simulink model "pmsm_summer_last"  (R2014a)
settings: Solver=ode23t  StartTime=0.0  StopTime=3  RelTol=1e-3
undefined symbols (not defined in the file or in its folder): sigbuilder_block
libraries: powerlib x6, powerlib_extras x3, simulink x1
settings Model: Creator=Andrew  LastModifiedBy=Administrator
settings DataIOCC: SignalLoggingSaveFormat=ModelDataLogs
settings OptimizationCC: ExpressionDepthLimit=2147483647
settings DebuggingCC: UnderspecifiedInitializationDetection=Classic  FcnCallInpInsideContextMsg=UseLocalSettings  StateNameClashWarn=warning
settings GRTTargetCC: CombineOutputUpdateFcns=off  GRTInterface=on

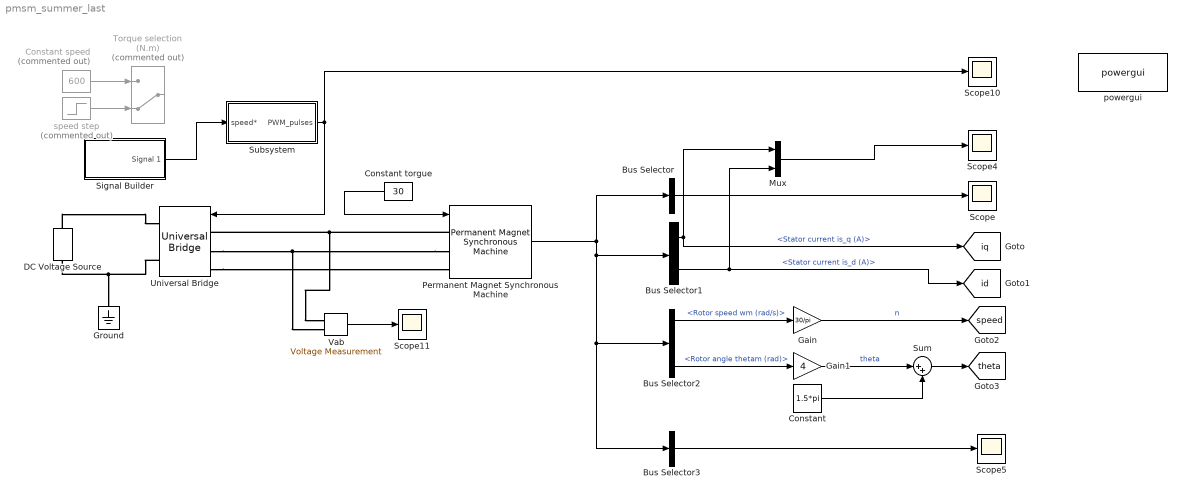
== system pmsm_summer_last ==
  Bus Selector : BusSelector  OutputSignals=Stator current is_a (A),Stator current is_b (A),Stator current is_c (A)  OutputAsBus=on
  Bus Selector1 : BusSelector  OutputSignals=Stator current is_q (A),Stator current is_d (A)
  Bus Selector2 : BusSelector  OutputSignals=Rotor speed wm (rad/s),Electromagnetic torque Te (N*m),Rotor angle thetam (rad)
  Bus Selector3 : BusSelector  OutputSignals=Stator voltage Vs_q (V),Stator voltage Vs_d (V)  OutputAsBus=on
  Constant : Constant  Value=1.5*pi
  Constant speed : Constant  Commented=on  Value=600
  Constant torgue : Constant  Value=30
  DC Voltage Source : powerlib/Electrical Sources/DC Voltage Source  Amplitude=300  Measurements=None
  Gain : Gain  Gain=30/pi
  Gain1 : Gain  Gain=4
  Ground : powerlib/Elements/Ground  LConnTagsString=a
  Mux : Mux  Inputs=2
  Permanent Magnet Synchronous Machine : powerlib/Machines/Permanent Magnet Synchronous Machine  NbPhases=3  FluxDistribution=Sinusoidal  RotorType=Round  MechanicalLoad=Torque Tm  PresetModel=No  ShowDetailedParameters=on  MeasurementBus=off  Resistance=2.8750  Inductance=8.5e-3  dqInductances=[8.5e-3,8.5e-3]  La=0.000835  MachineConstant=Flux linkage established by magnets (V.s)  Flux=0.175  VoltageCst=126.966  TorqueCst=1.05  Flat=120  Mechanical=[0.0008 0.001 4]  PolePairs=4  InitialConditions=[0,0, 0,0]  InitialConditions5ph=[0 0 0 0 0 0]  TsPowergui=0  TsBlock=-1  RefAngle=90 degrees behind phase A axis (modified Park)
  Scope{,4..5,10..11} (5 alike) : Scope
      Scope settings: YMin=-11  YMax=10
      Scope10 settings: TickLabels=on  YMin=0  YMax=1  SaveName=ScopeData6
      Scope11 settings: YMin=-350  YMax=350  SaveName=ScopeData8
      Scope4 settings: YMin=-0.5  YMax=5.25  SaveName=ScopeData4
      Scope5 settings: YMin=-200  YMax=225  SaveName=ScopeData5
  Signal Builder : Subsystem  Tag=STV Subsys  LoadFcn=sigbuilder_block('load');  StartFcn=sigbuilder_block('start');  StopFcn=sigbuilder_block('stop');  ClipboardFcn=sigbuilder_block('clipboard');  mask(Sigbuilder block){}
      mask help: Simulink:masks:SigbuilderBlock_MD
      mask init:
      | if ~strcmp(get_param(bdroot(gcbh),'SimulationStatus'),'stopped') tuvar = sigbuilder_block('maskInit'); end
      settings: CopyFcn=sigbuilder_block('copy');  DeleteFcn=sigbuilder_block('delete');  ModelCloseFcn=sigbuilder_block('modelClose');  PreSaveFcn=sigbuilder_block('preSave');  PauseFcn=sigbuilder_block('pause');  ContinueFcn=sigbuilder_block('continue');  NameChangeFcn=sigbuilder_block('namechange');  OpenFcn=sigbuilder_block('open',[295.5 114.75 550.5 393.75 ]);  CloseFcn=sigbuilder_block('close');
      mask Display: plot(0, 0, 100, 100,[2, 2, 32, 32, 2], [68, 8, 8, 68, 68],[32, 2], [38, 38], [32, 19, 2],[53, 60, 44], [32, 17, 17, 2],[16, 16, 31, 31]);txt = getActiveGroup(gcbh);text(2, 100, txt,'verticalAlignment', 'top');
  Subsystem : Subsystem
  Sum : Sum  Inputs=|++
  Torque selection (N.m) : ManualSwitch  Commented=on  CurrentSetting=0
  Universal Bridge : powerlib/Power Electronics/Universal Bridge  Arms=3  SnubberResistance=1e5  SnubberCapacitance=inf  Device=IGBT / Diodes  Ron=1e-3  Lon=0  ForwardVoltages="[  0  0  ]"  ForwardVoltage=0  GTOparameters=[ 10e-6 , 20e-6 ]  IGBTparameters=[ 1e-6 , 2e-6 ]  Measurements=None  Measurements_2=None  converterType=Rectifier
  Vab : powerlib/Measurements/Voltage Measurement  PhasorSimulation=off  OutputType=Complex  PSBequivalent=0
  powergui : powerlib/powergui  Priority=2  SimulationMode=Discrete  SolverType=Tustin  SampleTime=5e-6  frequency=60  SPID=off  DisableSnubberDevices=off  DisableRonSwitches=off  DisableVfSwitches=off  SwTol=0  Interpol=off  DisplayEquations=off  Ts=0  methode=off  frequencyindice=0  Pbase=100e6  ErrMax=1e-4  Iterations=50  UnitsV=kV  UnitsW=MW  FunctionMessages=off  echomessages=off  HookPort=off  EnableUseOfTLC=off  x0status=blocks  RestoreLinks=warning  ResistiveCurrentMeasurement=off  Frange=[0:2:500]  Ylog=off  Xlog=on  ShowGrid=off  save=off  variable=ZData  structure=0  ZoomFFT=on  StartTime=0.0  cycles=1  DisplayStyle=1  fundamental=60  FreqAxis=off  MaxFrequency=1000  frequencyindicesteady=1  RmsSteady=1  display=off
  speed step : Step  Commented=on  Time=0.5  Before=-100  After=100  SampleTime=0
  tag scope: id=global, iq=global, speed=global, theta=global
  wires:
  Constant torgue/1 -> Permanent Magnet Synchronous Machine/1
  Permanent Magnet Synchronous Machine/1 -> Bus Selector/1, Bus Selector1/1, Bus Selector2/1, Bus Selector3/1
  Bus Selector/1 -> Scope/1
  Bus Selector1/1 -> [iq], Mux/1  "<Stator current is_q (A)>"
  Bus Selector1/2 -> Mux/2, [id]  "<Stator current is_d (A)>"
  Bus Selector2/1 -> Gain/1  "<Rotor speed wm (rad/s)>"
  Bus Selector2/3 -> Gain1/1  "<Rotor angle thetam (rad)>"
  Gain/1 -> [speed]  "n"
  Gain1/1 -> Sum/1  "theta"
  Mux/1 -> Scope4/1
  Bus Selector3/1 -> Scope5/1
  Subsystem/1(PWM_pulses) -> Universal Bridge/1, Scope10/1
  Vab/1 -> Scope11/1
  speed step/1 -> Torque selection (N.m)/2
  Constant speed/1 -> Torque selection (N.m)/1
  Sum/1 -> [theta]
  Constant/1 -> Sum/2
  Signal Builder/1(Signal 1) -> Subsystem/1(speed*)
  connections:
  DC Voltage Source/RConn1 -- Universal Bridge/RConn1
  Universal Bridge/RConn2 -- DC Voltage Source/LConn1 -- Ground/LConn1
  Permanent Magnet Synchronous Machine/LConn1 -- Universal Bridge/LConn1 -- Vab/LConn1
  Permanent Magnet Synchronous Machine/LConn2 -- Universal Bridge/LConn2 -- Vab/LConn2
  Universal Bridge/LConn3 -- Permanent Magnet Synchronous Machine/LConn3

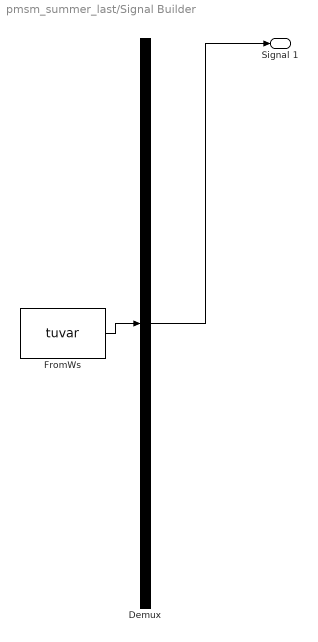
== system pmsm_summer_last/Signal Builder ==
  Demux : Demux  Tag=STV Demux  Outputs=1
  FromWs : FromWorkspace  Tag=STV FromWs  VariableName=tuvar  SampleTime=0
      SigBuilderData=|
      | common.afterFinalStr = 'Extrapolate'
      | common.sampleTime = 0
      | dataSet.timeRange = [0 10]
      | dataSet.name = 'Group 1'
      | sbobj.Groups.Name = 'Group 1'
      | sbobj.Groups.Signals.Name = 'Signal 1'
      | sbobj.Groups.Signals.XData = [0 1.02 1.02 2 2 10]
      | sbobj.Groups.Signals.YData = [0 0 100 100 -200 -200]
  Signal 1 : Outport  Tag=STV Outport
  wires:
  Demux/1 -> Signal 1/1
  FromWs/1 -> Demux/1

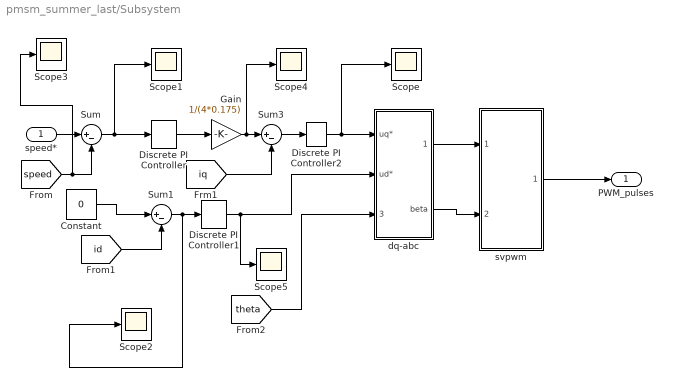
== system pmsm_summer_last/Subsystem ==
  speed* : Inport
  Constant : Constant  Value=0
  Discrete PI Controller : powerlib_extras/Discrete  Control Blocks/Discrete PI Controller  Kp=2.6  Ki=60  Par_Limits=[30 -30]  Init=0  Ts=5e-6
  Discrete PI Controller1 : powerlib_extras/Discrete  Control Blocks/Discrete PI Controller  Kp=10  Ki=1000  Par_Limits=[1e6 -1e6]  Init=0  Ts=5e-6
  Discrete PI Controller2 : powerlib_extras/Discrete  Control Blocks/Discrete PI Controller  Kp=3  Ki=100  Par_Limits=[1e6 -1e6]  Init=0  Ts=5e-6
  Gain : Gain  Gain=1/(4*0.175)
  Scope{,1..5} (6 alike) : Scope
      Scope settings: YMin=-300  YMax=300  SaveName=ScopeData7
      Scope1 settings: YMin=-300  YMax=300  SaveName=ScopeData3
      Scope2 settings: YMin=-300  YMax=300  SaveName=ScopeData9
      Scope3 settings: YMin=98.25  YMax=102  SaveName=ScopeData10
      Scope4 settings: YMin=19  YMax=37  SaveName=ScopeData11
      Scope5 settings: YMin=-300  YMax=300  SaveName=ScopeData12
  Sum : Sum  Inputs=|+-
  Sum1 : Sum  Inputs=|+-
  Sum3 : Sum  Inputs=|+-
  dq-abc : Subsystem
  svpwm : Subsystem
  PWM_pulses : Outport
  wires:
  speed*/1 -> Sum/1
  [speed] -> Scope3/1, Sum/2
  Sum/1 -> Scope1/1, Discrete PI Controller/1
  Discrete PI Controller/1 -> Gain/1
  Sum3/1 -> Discrete PI Controller2/1
  [iq] -> Sum3/2
  Discrete PI Controller2/1 -> Scope/1, dq-abc/1(uq*)
  [theta] -> dq-abc/3(theta)
  dq-abc/1(alpha) -> svpwm/1(alpha1)
  dq-abc/2(beta) -> svpwm/2(beta1)
  svpwm/1(pluses) -> PWM_pulses/1
  Gain/1 -> Scope4/1, Sum3/1
  Sum1/1 -> Scope2/1, Discrete PI Controller1/1
  Discrete PI Controller1/1 -> Scope5/1, dq-abc/2(ud*)
  [id] -> Sum1/2
  Constant/1 -> Sum1/1

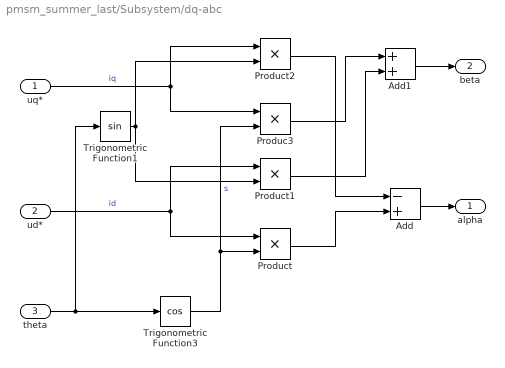
== system pmsm_summer_last/Subsystem/dq-abc ==
  uq* : Inport
  ud* : Inport  Port=2
  theta : Inport  Port=3
  Add : Sum  Inputs=-+
  Add1 : Sum
  Produc3 : Product  RndMeth=Zero
  Product : Product  RndMeth=Zero
  Product1 : Product  RndMeth=Zero
  Product2 : Product  RndMeth=Zero
  Trigonometric Function1 : Trigonometry
  Trigonometric Function3 : Trigonometry  Operator=cos
  alpha : Outport
  beta : Outport  Port=2
  wires:
  theta/1 -> Trigonometric Function1/1, Trigonometric Function3/1
  uq*/1 -> Product2/1, Produc3/1  "iq"
  ud*/1 -> Product1/1, Product/1  "id"
  Trigonometric Function1/1 -> Product1/2, Product2/2
  Trigonometric Function3/1 -> Product/2, Produc3/2  "s"
  Product2/1 -> Add/1
  Product/1 -> Add/2
  Add/1 -> alpha/1
  Add1/1 -> beta/1
  Product1/1 -> Add1/2
  Produc3/1 -> Add1/1

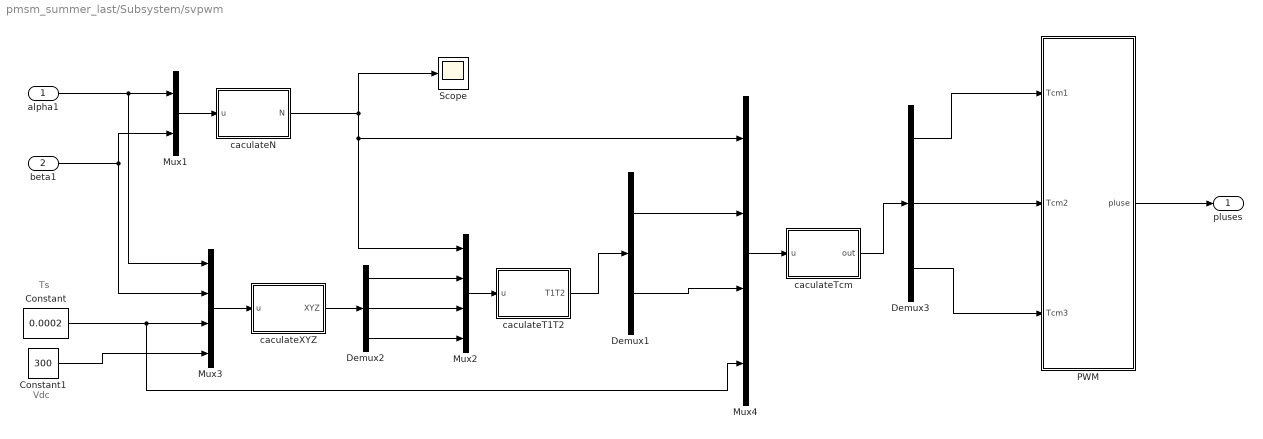
== system pmsm_summer_last/Subsystem/svpwm ==
  note: Vdc
  note: Ts
  alpha1 : Inport
  beta1 : Inport  Port=2
  Constant : Constant  Value=0.0002
  Constant1 : Constant  Value=300
  Demux1 : Demux  Outputs=2
  Demux2 : Demux  Outputs=3
  Demux3 : Demux  Outputs=3
  Mux1 : Mux  Inputs=2
  Mux2 : Mux
  Mux3 : Mux
  Mux4 : Mux
  PWM : Subsystem
  Scope : Scope
      settings: YMin=1  YMax=6  SaveName=ScopeData2
  caculateN : MATLAB Function  TreatAsAtomicUnit=on
  caculateT1T2 : MATLAB Function  TreatAsAtomicUnit=on
  caculateTcm : MATLAB Function  TreatAsAtomicUnit=on
  caculateXYZ : MATLAB Function  TreatAsAtomicUnit=on
  pluses : Outport
  wires:
  alpha1/1 -> Mux3/1, Mux1/1
  beta1/1 -> Mux3/2, Mux1/2
  Constant/1 -> Mux4/4, Mux3/3
  caculateN/1(N) -> Mux2/1, Mux4/1, Scope/1
  PWM/1(pluse) -> pluses/1
  Mux1/1 -> caculateN/1(u)
  Mux3/1 -> caculateXYZ/1(u)
  caculateXYZ/1(XYZ) -> Demux2/1
  Constant1/1 -> Mux3/4
  Mux2/1 -> caculateT1T2/1(u)
  caculateT1T2/1(T1T2) -> Demux1/1
  Demux2/1 -> Mux2/2
  Demux2/2 -> Mux2/3
  Demux2/3 -> Mux2/4
  Mux4/1 -> caculateTcm/1(u)
  caculateTcm/1(out) -> Demux3/1
  Demux1/1 -> Mux4/2
  Demux1/2 -> Mux4/3
  Demux3/1 -> PWM/1(Tcm1)
  Demux3/2 -> PWM/2(Tcm2)
  Demux3/3 -> PWM/3(Tcm3)

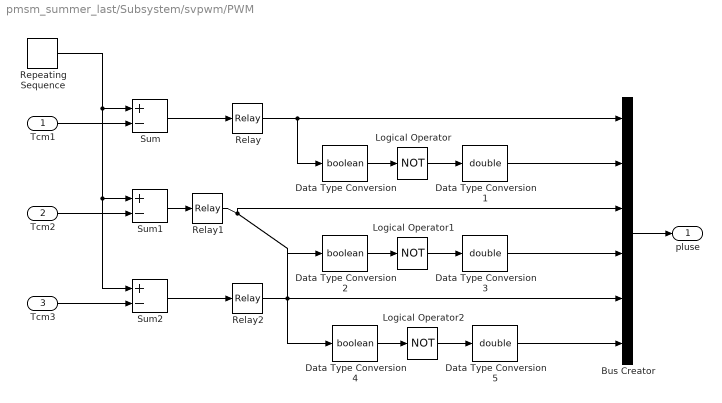
== system pmsm_summer_last/Subsystem/svpwm/PWM ==
  Tcm1 : Inport
  Tcm2 : Inport  Port=2
  Tcm3 : Inport  Port=3
  Bus Creator : BusCreator  Inputs=6
  Data Type Conversion : DataTypeConversion  OutDataTypeStr=boolean
  Data Type Conversion1 : DataTypeConversion  OutDataTypeStr=double
  Data Type Conversion2 : DataTypeConversion  OutDataTypeStr=boolean
  Data Type Conversion3 : DataTypeConversion  OutDataTypeStr=double
  Data Type Conversion4 : DataTypeConversion  OutDataTypeStr=boolean
  Data Type Conversion5 : DataTypeConversion  OutDataTypeStr=double
  Logical Operator : Logic  Operator=NOT  AllPortsSameDT=off  OutDataTypeStr=boolean
  Logical Operator1 : Logic  Operator=NOT  AllPortsSameDT=off  OutDataTypeStr=boolean
  Logical Operator2 : Logic  Operator=NOT  AllPortsSameDT=off  OutDataTypeStr=boolean
  Relay : Relay
  Relay1 : Relay
  Relay2 : Relay
  Repeating Sequence : simulink/Sources/Repeating Sequence  rep_seq_t=[0 0.0001 0.0002]  rep_seq_y=[0 0.0001 0]
  Sum : Sum  Inputs=+-
  Sum1 : Sum  Inputs=+-
  Sum2 : Sum  Inputs=+-
  pluse : Outport
  wires:
  Tcm1/1 -> Sum/2
  Repeating Sequence/1 -> Sum/1, Sum1/1, Sum2/1
  Tcm2/1 -> Sum1/2
  Tcm3/1 -> Sum2/2
  Sum/1 -> Relay/1
  Sum1/1 -> Relay1/1
  Sum2/1 -> Relay2/1
  Relay/1 -> Data Type Conversion/1, Bus Creator/1
  Data Type Conversion/1 -> Logical Operator/1
  Logical Operator/1 -> Data Type Conversion1/1
  Data Type Conversion2/1 -> Logical Operator1/1
  Logical Operator1/1 -> Data Type Conversion3/1
  Relay1/1 -> Data Type Conversion2/1, Bus Creator/3
  Data Type Conversion4/1 -> Logical Operator2/1
  Logical Operator2/1 -> Data Type Conversion5/1
  Data Type Conversion1/1 -> Bus Creator/2
  Data Type Conversion3/1 -> Bus Creator/4
  Data Type Conversion5/1 -> Bus Creator/6
  Bus Creator/1 -> pluse/1
  Relay2/1 -> Data Type Conversion4/1, Bus Creator/5

== matlab function pmsm_summer_last/Subsystem/svpwm/caculateXYZ ==
  data: u input; XYZ output
function XYZ = fcn(u)
Ua=u(1);
Ub=u(2);
Ts=u(3);     %daiding
Ud=u(4);       %daiding
X=sqrt(3)*Ub*Ts/Ud;
Y=(3*Ua+sqrt(3)*Ub)*Ts/(2*Ud);
Z=(-3*Ua+sqrt(3)*Ub)*Ts/(2*Ud);
XYZ=[X,Y,Z]';

== matlab function pmsm_summer_last/Subsystem/svpwm/caculateT1T2 ==
  data: u input; T1T2 output
function T1T2 = fcn(u)
N=u(1);
X=u(2);
Y=u(3);
Z=u(4);   
switch N
    case 1
        T1=Z;
        T2=Y;
    case 2
        T1=Y;
        T2=-X;
    case 3
        T1=-Z;
        T2=X;
    case 4
        T1=-X;
        T2=Z;
    case 5
        T1=X;
        T2=-Y;
    case 6
        T1=-Y;
        T2=-Z;
    otherwise
        T1=Z;
        T2=Y;
end
T1T2=[T1,T2]';

== matlab function pmsm_summer_last/Subsystem/svpwm/caculateN ==
  data: u input; N output
function N = fcn(u)
Ua=u(1);
Ub=u(2);
In=[Ua;Ub];
T=[0,1;sqrt(3),-1;-sqrt(3),-1];
Out=T*In;
if Out(1)>0
    A=1;
else
    A=0;
end
if Out(2)>0
    B=1;
else
    B=0;
end
if Out(3)>0
    C=1;
else
    C=0;
end
N=A+2*B+4*C;

== matlab function pmsm_summer_last/Subsystem/svpwm/caculateTcm ==
  data: u input; out output
function out = fcn(u)
N=u(1);
T1=u(2);
T2=u(3);
Ts=u(4);
if T1 + T2>Ts
    T3=T1;
    T1=T1*Ts/(T1+T2);
    T2=T2*Ts/(T3+T2);
end
T0=(Ts-T1-T2)/2;
Ta=1/2*T0;
Tb=1/2*T0+1/2*T1;
Tc=1/2*T0+1/2*T1+1/2*T2;

switch N
    case 1
        out=[Tb,Ta,Tc]';
    case 2
        out=[Ta,Tc,Tb]';
    case 3
        out=[Ta,Tb,Tc]';
    case 4
        out=[Tc,Tb,Ta]';
    case 5
        out=[Tc,Ta,Tb]';
    case 6
        out=[Tb,Tc,Ta]';
    otherwise
        out=[Tb,Ta,Tc]';
end
